simulink model "FBFunctions"  (R2018b)
settings: Solver=VariableStepAuto  StartTime=0.0  StopTime=10.0  RelTol=1e-3
libraries: library x32
settings Model: Creator=hiterd  LastModifiedBy=gauthamsm
settings SFSimCC: SimUseLocalCustomCode=off
settings RTWCC: RTWUseLocalCustomCode=off

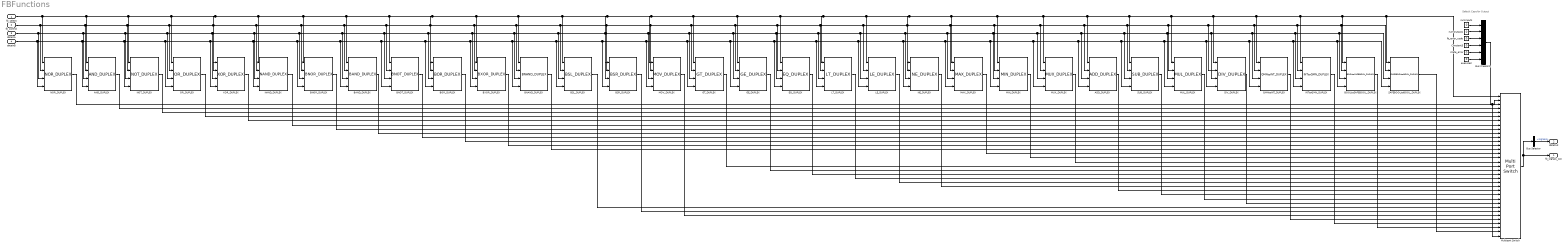
== system FBFunctions ==
  note: Default Case for Output
  fb_select : Inport  OutDataTypeStr=int32
  fb_control : Inport  Port=2  OutDataTypeStr=Bus: fb_control
  dataInA : Inport  Port=3  OutDataTypeStr=int32
  dataInB : Inport  Port=4  OutDataTypeStr=int32
  ADD_DUPLEX : library/ADD_DUPLEX  SystemSampleTime=-1  VariantControl=MUX_FB
  AND_DUPLEX : library/AND_DUPLEX  SystemSampleTime=-1  VariantControl=MUX_FB
  BAND_DUPLEX : library/BAND_DUPLEX  SystemSampleTime=-1  VariantControl=MUX_FB
  BNAND_DUPLEX : library/BNAND_DUPLEX  SystemSampleTime=-1  VariantControl=MUX_FB
  BNOR_DUPLEX : library/BNOR_DUPLEX  SystemSampleTime=-1  VariantControl=MUX_FB
  BNOT_DUPLEX : library/BNOT_DUPLEX  SystemSampleTime=-1  VariantControl=MUX_FB
  BOOLtoSAFEBOOL_DUPLEX : library/BOOLtoSAFEBOOL_DUPLEX  SystemSampleTime=-1  VariantControl=MUX_FB
  BOR_DUPLEX : library/BOR_DUPLEX  SystemSampleTime=-1  VariantControl=MUX_FB
  BSL_DUPLEX : library/BSL_DUPLEX  SystemSampleTime=-1  VariantControl=MUX_FB
  BSR_DUPLEX : library/BSR_DUPLEX  SystemSampleTime=-1  VariantControl=MUX_FB
  BXOR_DUPLEX : library/BXOR_DUPLEX  SystemSampleTime=-1  VariantControl=MUX_FB
  Bus Creator1 : BusCreator  Inputs=6  OutDataTypeStr=Bus: fb_functions_out
  Bus Selector : BusSelector  OutputSignals=signal4
  Constant3 : Constant  Value=0  OutDataTypeStr=int32  SampleTime=-1
  DIV_DUPLEX : library/DIV_DUPLEX  SystemSampleTime=-1  VariantControl=MUX_FB
  EQ_DUPLEX : library/EQ_DUPLEX  SystemSampleTime=-1  VariantControl=MUX_FB
  GE_DUPLEX : library/GE_DUPLEX  SystemSampleTime=-1  VariantControl=MUX_FB
  GT_DUPLEX : library/GT_DUPLEX  SystemSampleTime=-1  VariantControl=MUX_FB
  INTtoQMN_DUPLEX : library/INTtoQMN_DUPLEX  SystemSampleTime=-1  VariantControl=MUX_FB
  LE_DUPLEX : library/LE_DUPLEX  SystemSampleTime=-1  VariantControl=MUX_FB
  LT_DUPLEX : library/LT_DUPLEX  SystemSampleTime=-1  VariantControl=MUX_FB
  MAX_DUPLEX : library/MAX_DUPLEX  SystemSampleTime=-1  VariantControl=MUX_FB
  MIN_DUPLEX : library/MIN_DUPLEX  SystemSampleTime=-1  VariantControl=MUX_FB
  MOV_DUPLEX : library/MOV_DUPLEX  SystemSampleTime=-1  VariantControl=MUX_FB
  MUL_DUPLEX : library/MUL_DUPLEX  SystemSampleTime=-1  VariantControl=MUX_FB
  MUX_DUPLEX : library/MUX_DUPLEX  SystemSampleTime=-1  VariantControl=MUX_FB
  Multiport Switch : MultiPortSwitch  DataPortOrder=Zero-based contiguous  Inputs=33  DataPortForDefault=Additional data port  zeroidx=on  OutDataTypeStr=Inherit: Inherit via back propagation
  NAND_DUPLEX : library/NAND_DUPLEX  SystemSampleTime=-1  VariantControl=MUX_FB
  NE_DUPLEX : library/NE_DUPLEX  SystemSampleTime=-1  VariantControl=MUX_FB
  NOR_DUPLEX : library/NOR_DUPLEX  SystemSampleTime=-1  VariantControl=MUX_FB
  NOT_DUPLEX : library/NOT_DUPLEX  SystemSampleTime=-1  VariantControl=MUX_FB
  OR_DUPLEX : library/OR_DUPLEX  SystemSampleTime=-1  VariantControl=MUX_FB
  QMNtoINT_DUPLEX : library/QMNtoINT_DUPLEX  SystemSampleTime=-1  VariantControl=MUX_FB
  SAFEBOOLtoBOOL_DUPLEX : library/SAFEBOOLtoBOOL_DUPLEX  SystemSampleTime=-1  VariantControl=MUX_FB
  SUB_DUPLEX : library/SUB_DUPLEX  SystemSampleTime=-1  VariantControl=MUX_FB
  XOR_DUPLEX : library/XOR_DUPLEX  SystemSampleTime=-1  VariantControl=MUX_FB
  executed : Constant  Value=0  OutDataTypeStr=boolean  SampleTime=-1
  fb_error_code : Constant  Value=0  OutDataTypeStr=uint32  SampleTime=-1
  numInputs : Constant  Value=0  OutDataTypeStr=uint8  SampleTime=-1
  numOutputs : Constant  Value=0  OutDataTypeStr=uint8  SampleTime=-1
  state_error : Constant  Value=0  OutDataTypeStr=boolean  SampleTime=-1
  fb_signals_out : Outport  OutDataTypeStr=Bus: fb_functions_out
  dataOut : Outport  Port=2
  wires:
  Multiport Switch/1 -> fb_signals_out/1, Bus Selector/1
  Bus Selector/1 -> dataOut/1  "<signal4>"
  Bus Creator1/1 -> Multiport Switch/35, Multiport Switch/2
  numInputs/1 -> Bus Creator1/1
  executed/1 -> Bus Creator1/6
  state_error/1 -> Bus Creator1/5
  Constant3/1 -> Bus Creator1/4
  fb_error_code/1 -> Bus Creator1/3
  numOutputs/1 -> Bus Creator1/2
  fb_select/1 -> NOR_DUPLEX/1, AND_DUPLEX/1, NOT_DUPLEX/1, OR_DUPLEX/1, XOR_DUPLEX/1, NAND_DUPLEX/1, BNOR_DUPLEX/1, BAND_DUPLEX/1, BNOT_DUPLEX/1, BOR_DUPLEX/1, BXOR_DUPLEX/1, BNAND_DUPLEX/1, BSL_DUPLEX/1, BSR_DUPLEX/1, MOV_DUPLEX/1, GT_DUPLEX/1, GE_DUPLEX/1, EQ_DUPLEX/1, LT_DUPLEX/1, LE_DUPLEX/1, NE_DUPLEX/1, MAX_DUPLEX/1, MIN_DUPLEX/1, MUX_DUPLEX/1, ADD_DUPLEX/1, SUB_DUPLEX/1, MUL_DUPLEX/1, DIV_DUPLEX/1, QMNtoINT_DUPLEX/1, INTtoQMN_DUPLEX/1, BOOLtoSAFEBOOL_DUPLEX/1, SAFEBOOLtoBOOL_DUPLEX/1, Multiport Switch/1
  fb_control/1 -> NOR_DUPLEX/2, AND_DUPLEX/2, NOT_DUPLEX/2, OR_DUPLEX/2, XOR_DUPLEX/2, NAND_DUPLEX/2, BNOR_DUPLEX/2, BAND_DUPLEX/2, BNOT_DUPLEX/2, BOR_DUPLEX/2, BXOR_DUPLEX/2, BNAND_DUPLEX/2, BSL_DUPLEX/2, BSR_DUPLEX/2, MOV_DUPLEX/2, GT_DUPLEX/2, GE_DUPLEX/2, EQ_DUPLEX/2, LT_DUPLEX/2, LE_DUPLEX/2, NE_DUPLEX/2, MAX_DUPLEX/2, MIN_DUPLEX/2, MUX_DUPLEX/2, ADD_DUPLEX/2, SUB_DUPLEX/2, MUL_DUPLEX/2, QMNtoINT_DUPLEX/2, INTtoQMN_DUPLEX/2, BOOLtoSAFEBOOL_DUPLEX/2, SAFEBOOLtoBOOL_DUPLEX/2, DIV_DUPLEX/2
  dataInA/1 -> NOR_DUPLEX/3, AND_DUPLEX/3, NOT_DUPLEX/3, OR_DUPLEX/3, XOR_DUPLEX/3, NAND_DUPLEX/3, BNOR_DUPLEX/3, BAND_DUPLEX/3, BNOT_DUPLEX/3, BOR_DUPLEX/3, BXOR_DUPLEX/3, BNAND_DUPLEX/3, BSL_DUPLEX/3, BSR_DUPLEX/3, MOV_DUPLEX/3, GT_DUPLEX/3, GE_DUPLEX/3, EQ_DUPLEX/3, LT_DUPLEX/3, LE_DUPLEX/3, NE_DUPLEX/3, MAX_DUPLEX/3, MIN_DUPLEX/3, MUX_DUPLEX/3, ADD_DUPLEX/3, SUB_DUPLEX/3, MUL_DUPLEX/3, QMNtoINT_DUPLEX/3, INTtoQMN_DUPLEX/3, BOOLtoSAFEBOOL_DUPLEX/3, SAFEBOOLtoBOOL_DUPLEX/3, DIV_DUPLEX/3
  dataInB/1 -> NOR_DUPLEX/4, AND_DUPLEX/4, NOT_DUPLEX/4, OR_DUPLEX/4, XOR_DUPLEX/4, NAND_DUPLEX/4, BNOR_DUPLEX/4, BAND_DUPLEX/4, BNOT_DUPLEX/4, BOR_DUPLEX/4, BXOR_DUPLEX/4, BNAND_DUPLEX/4, BSL_DUPLEX/4, BSR_DUPLEX/4, MOV_DUPLEX/4, GT_DUPLEX/4, GE_DUPLEX/4, EQ_DUPLEX/4, LT_DUPLEX/4, LE_DUPLEX/4, NE_DUPLEX/4, MAX_DUPLEX/4, MIN_DUPLEX/4, MUX_DUPLEX/4, ADD_DUPLEX/4, SUB_DUPLEX/4, MUL_DUPLEX/4, QMNtoINT_DUPLEX/4, INTtoQMN_DUPLEX/4, BOOLtoSAFEBOOL_DUPLEX/4, SAFEBOOLtoBOOL_DUPLEX/4, DIV_DUPLEX/4
  DIV_DUPLEX/1 -> Multiport Switch/27
  MUL_DUPLEX/1 -> Multiport Switch/26
  SUB_DUPLEX/1 -> Multiport Switch/25
  ADD_DUPLEX/1 -> Multiport Switch/24
  MUX_DUPLEX/1 -> Multiport Switch/17
  MIN_DUPLEX/1 -> Multiport Switch/16
  MAX_DUPLEX/1 -> Multiport Switch/15
  NE_DUPLEX/1 -> Multiport Switch/23
  LE_DUPLEX/1 -> Multiport Switch/22
  LT_DUPLEX/1 -> Multiport Switch/21
  EQ_DUPLEX/1 -> Multiport Switch/20
  GE_DUPLEX/1 -> Multiport Switch/19
  GT_DUPLEX/1 -> Multiport Switch/18
  MOV_DUPLEX/1 -> Multiport Switch/30
  BSR_DUPLEX/1 -> Multiport Switch/29
  BSL_DUPLEX/1 -> Multiport Switch/28
  BNAND_DUPLEX/1 -> Multiport Switch/14
  BXOR_DUPLEX/1 -> Multiport Switch/13
  BOR_DUPLEX/1 -> Multiport Switch/12
  BNOT_DUPLEX/1 -> Multiport Switch/11
  BAND_DUPLEX/1 -> Multiport Switch/10
  BNOR_DUPLEX/1 -> Multiport Switch/9
  NAND_DUPLEX/1 -> Multiport Switch/8
  XOR_DUPLEX/1 -> Multiport Switch/7
  OR_DUPLEX/1 -> Multiport Switch/6
  NOT_DUPLEX/1 -> Multiport Switch/5
  AND_DUPLEX/1 -> Multiport Switch/4
  NOR_DUPLEX/1 -> Multiport Switch/3
  QMNtoINT_DUPLEX/1 -> Multiport Switch/31
  INTtoQMN_DUPLEX/1 -> Multiport Switch/32
  BOOLtoSAFEBOOL_DUPLEX/1 -> Multiport Switch/33
  SAFEBOOLtoBOOL_DUPLEX/1 -> Multiport Switch/34
